simulink model "whole"  (R2022b)
settings: Solver=VariableStepAuto  StartTime=0.0  StopTime=7  FixedStep=1e-4  RelTol=1e-3
values from neighbouring files (symbols this model uses):
  ad = [ax' ay' az']    [whole_main.m]
  dt = 0.005    [whole_main.m]
  J = diag([0.082,0.0845,0.1377])    [whole_main.m]
  K = lqr(sys,Q,R)    [whole_main.m]
  kv = 5.6    [whole_main.m]
  kx = 16    [whole_main.m]
  m = 4.34    [whole_main.m]
  pd = [x' y' z']    [whole_main.m]
  psi_d = 0.1*t'    [whole_main.m]
  vd = [vx' vy' vz']    [whole_main.m]
libraries: shared6dof x1, aerolibutil x1
settings Model: Creator=zzy  LastModifiedBy=zzy
settings DataIOCC: ReturnWorkspaceOutputs=off

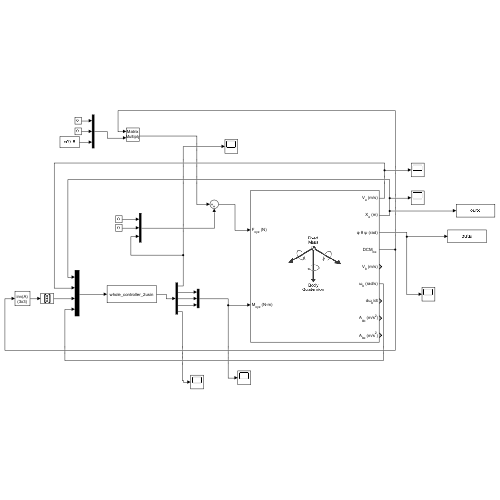
[thumbnail: Simulink's stored preview of the top-level diagram]
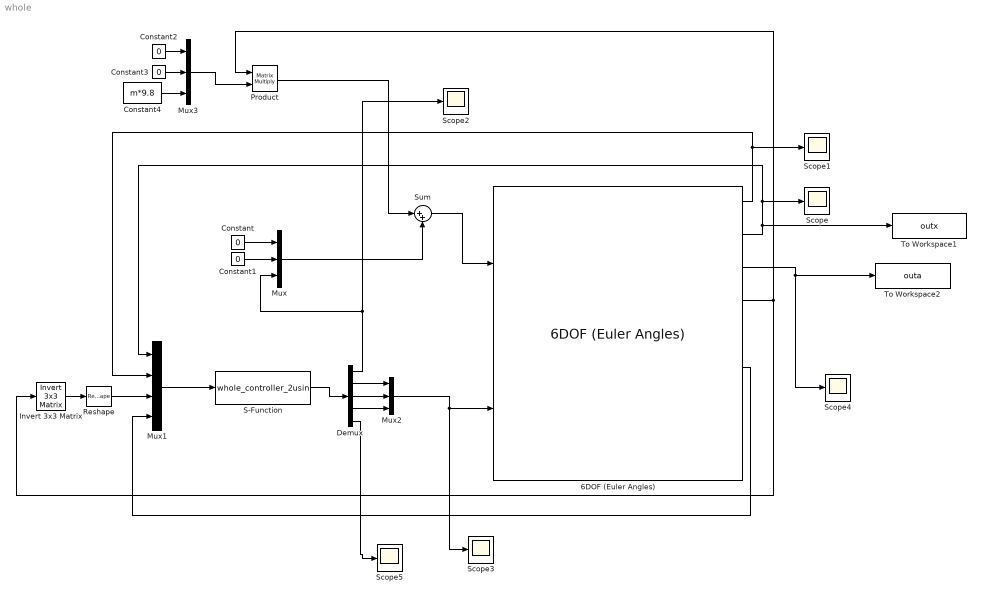
== system whole ==
  6DOF (Euler Angles) : shared6dof/6DOF (Euler Angles)  units=Metric (MKS)  mtype=Fixed  rep=Quaternion  xme_0=[0 0 0]  Vm_0=[0 0 0]  eul_0=[0 0 0]  pm_0=[0 0 0]  mass_0=m  mass_e=0.5  mass_f=2.0  inertia=J  inertia_e=eye(3)  inertia_f=2*eye(3)  k_quat=1.0  vre_flag=on  abi_flag=on  aMode=0  xme_statename=''  Vm_statename=''  eul_statename=''  quat_statename=''  pm_statename=''  mass_statename=''
  Constant{,1..3} (4 alike) : Constant  Value=0
  Constant4 : Constant  Value=m*9.8
  Demux : Demux  Outputs=5
  Invert 3x3 Matrix : aerolibutil/Invert  3x3 Matrix
  Mux : Mux  Inputs=3
  Mux1 : Mux
  Mux2 : Mux  Inputs=3
  Mux3 : Mux  Inputs=3
  Product : Product  Multiplication=Matrix(*)
  Reshape : Reshape  OutputDimensionality=Column vector (2-D)
  S-Function : S-Function  FunctionName=whole_controller_2usin  Parameters=dt,pd,vd,ad,psi_d,m,J,kx,kv,K  SFunctionDeploymentMode=off  EnableBusSupport=off
  Scope{,1..5} (6 alike) : Scope
  Sum : Sum  Inputs=|++
  To Workspace1 : ToWorkspace  VariableName=outx  SampleTime=-1
      settings: Save2DSignal=2-D array (concatenate along first dimension)
  To Workspace2 : ToWorkspace  VariableName=outa  SampleTime=-1
      settings: Save2DSignal=2-D array (concatenate along first dimension)
  wires:
  Reshape/1 -> Mux1/3
  Mux1/1 -> S-Function/1
  6DOF (Euler Angles)/4 -> Product/1, Invert 3x3 Matrix/1
  6DOF (Euler Angles)/3 -> Scope4/1, To Workspace2/1
  Constant/1 -> Mux/1
  6DOF (Euler Angles)/6 -> Mux1/4
  Constant1/1 -> Mux/2
  S-Function/1 -> Demux/1
  Demux/1 -> Mux/3, Scope2/1
  Demux/2 -> Mux2/1
  Demux/3 -> Mux2/2
  Demux/4 -> Mux2/3
  6DOF (Euler Angles)/2 -> To Workspace1/1, Scope/1, Mux1/1
  6DOF (Euler Angles)/1 -> Scope1/1, Mux1/2
  Invert 3x3 Matrix/1 -> Reshape/1
  Mux2/1 -> Scope3/1, 6DOF (Euler Angles)/2
  Constant3/1 -> Mux3/2
  Constant2/1 -> Mux3/1
  Constant4/1 -> Mux3/3
  Mux3/1 -> Product/2
  Product/1 -> Sum/1
  Mux/1 -> Sum/2
  Sum/1 -> 6DOF (Euler Angles)/1
  Demux/5 -> Scope5/1
